simulink model "pure_pursuit"  (R2019b)
settings: Solver=FixedStepAuto  StartTime=0.0  StopTime=10.0  RelTol=1e-3
undefined symbols (not defined in the file): end_location, start_location
libraries: robotlib x6, robotalgslib x1

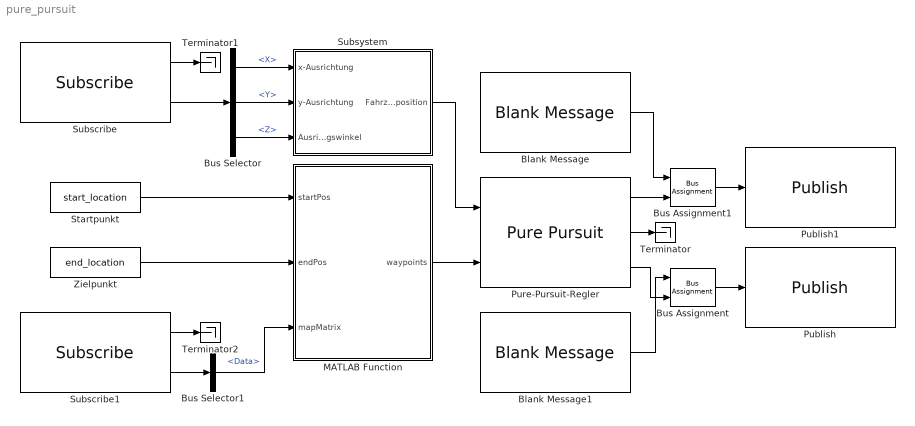
== system pure_pursuit ==
  Blank Message : robotlib/Blank Message  messageClass=Message  entityType=std_msgs/Float32  messageType=std_msgs/Float32  SampleTime=inf
  Blank Message1 : robotlib/Blank Message  messageClass=Message  entityType=std_msgs/Int16  messageType=std_msgs/Int16  SampleTime=inf
  Bus Assignment : BusAssignment  AssignedSignals=Data
  Bus Assignment1 : BusAssignment  AssignedSignals=Data
  Bus Selector : BusSelector  OutputSignals=X,Y,Z
  Bus Selector1 : BusSelector  OutputSignals=Data
  MATLAB Function : MATLAB Function  TreatAsAtomicUnit=on
  Publish : robotlib/Publish  topicSource=Specify your own  topic=/ctl_servoAngle  messageType=std_msgs/Float32  messageQueueLength=1
  Publish1 : robotlib/Publish  topicSource=Specify your own  topic=/ctl_motorRpm  messageType=std_msgs/Int16  messageQueueLength=1
  Pure-Pursuit-Regler : robotalgslib/Pure Pursuit  DesiredLinearVelocity=0.1  MaxAngularVelocity=1.0  LookaheadDistance=1.0  TargetDirPort=on  SimulateUsing=Code generation
  Startpunkt : Constant  Value=start_location
  Subscribe : robotlib/Subscribe  topicSource=Specify your own  topic=/trj_vehiclePose  messageType=geometry_msgs/Point  sampleTime=-1  messageQueueLength=1
  Subscribe1 : robotlib/Subscribe  topicSource=Specify your own  topic=/trj_roadMap  messageType=std_msgs/Float32MultiArray  sampleTime=-1  messageQueueLength=1
  Subsystem : Subsystem
  Terminator : Terminator
  Terminator1 : Terminator
  Terminator2 : Terminator
  Zielpunkt : Constant  Value=end_location
  wires:
  MATLAB Function/1(waypoints) -> Pure-Pursuit-Regler/2
  Zielpunkt/1 -> MATLAB Function/2(endPos)
  Startpunkt/1 -> MATLAB Function/1(startPos)
  Pure-Pursuit-Regler/3 -> Bus Assignment/2
  Bus Assignment/1 -> Publish/1
  Pure-Pursuit-Regler/1 -> Bus Assignment1/2
  Bus Assignment1/1 -> Publish1/1
  Blank Message/1 -> Bus Assignment1/1
  Blank Message1/1 -> Bus Assignment/1
  Pure-Pursuit-Regler/2 -> Terminator/1
  Subsystem/1(Fahrzeugposition) -> Pure-Pursuit-Regler/1
  Subscribe/2 -> Bus Selector/1
  Bus Selector/1 -> Subsystem/1(x-Ausrichtung)  "<X>"
  Bus Selector/2 -> Subsystem/2(y-Ausrichtung)  "<Y>"
  Bus Selector/3 -> Subsystem/3(Ausrichtungswinkel)  "<Z>"
  Subscribe/1 -> Terminator1/1
  Subscribe1/1 -> Terminator2/1
  Subscribe1/2 -> Bus Selector1/1
  Bus Selector1/1 -> MATLAB Function/3(mapMatrix)  "<Data>"

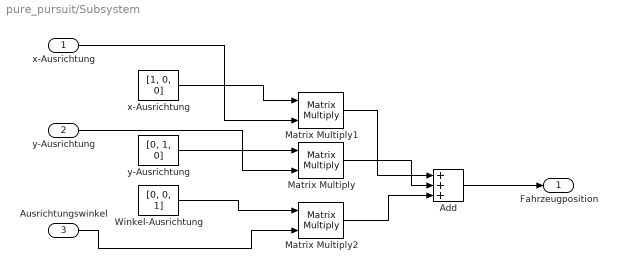
== system pure_pursuit/Subsystem ==
  x-Ausrichtung : Inport
  y-Ausrichtung : Inport  Port=2
  Ausrichtungswinkel : Inport  Port=3
  Add : Sum  Inputs=+++
  Matrix Multiply : Product  Multiplication=Matrix(*)
  Matrix Multiply1 : Product  Multiplication=Matrix(*)
  Matrix Multiply2 : Product  Multiplication=Matrix(*)
  Winkel-Ausrichtung : Constant  Value=[0, 0, 1]
  "x-Ausrichtung " : Constant  Value=[1, 0, 0]
  "y-Ausrichtung " : Constant  Value=[0, 1, 0]
  Fahrzeugposition : Outport
  wires:
  Matrix Multiply/1 -> Add/2
  x-Ausrichtung/1 -> Matrix Multiply1/2
  Matrix Multiply1/1 -> Add/1
  Winkel-Ausrichtung/1 -> Matrix Multiply2/1
  "y-Ausrichtung "/1 -> Matrix Multiply/1
  Matrix Multiply2/1 -> Add/3
  Ausrichtungswinkel/1 -> Matrix Multiply2/2
  "x-Ausrichtung "/1 -> Matrix Multiply1/1
  y-Ausrichtung/1 -> Matrix Multiply/2
  Add/1 -> Fahrzeugposition/1

== matlab function pure_pursuit/MATLAB Function ==
function waypoints = planning(startPos, endPos, mapMatrix)

persistent waypointsInternal
persistent prevStartPos
persistent prevEndPos

% Set constant parameters
maxNumNodes = 100;

% Initialize persistent variables that are used downstream
if isempty(prevStartPos)
    prevStartPos = startPos;
end

if isempty(prevEndPos)
    prevEndPos = endPos;
end

isNewPath = (~isequal(prevStartPos, startPos) || ~isequal(prevEndPos, endPos));

if isempty(waypointsInternal) || isNewPath
    % Two conditions in which waypoints must be set: they are not yet
    % initialized, or they are initialized, but the current start and end
    % do not match those used to generate the previous set of waypoints
    [waypointsInternal] = planPath(mapMatrix, maxNumNodes, startPos, endPos);
end

% Update the outputs
waypoints = waypointsInternal;

% Update the persistent variables that indicate previous state
prevStartPos = startPos;
prevEndPos = endPos;

%% Helper Function

function wayPoints = planPath(mapMatrix, maxNodes, startPos, endPos)
    
    % Create a probabilistic roadmap
    map = binaryOccupancyMap(mapMatrix);
    prm = mobileRobotPRM(map, maxNodes);
    
    % Find a path between two points
    xy = findpath(prm, startPos(:)', endPos(:)');
    wayPoints = repmat(endPos(:)', maxNodes, 1);
    
    % Number of nodes that are actually used
    numNodes = length(xy);
    wayPoints(1:numNodes,:) = xy;    

end

end
